simulink model "model_u2_x2"  (R2023b)
settings: Solver=VariableStepAuto  StartTime=0.0  StopTime=100.0  RelTol=1e-3
undefined symbols (not defined in the file or in its folder): a, alfa, beta, K, k, m, w_0, x_0, x_prim_0
settings Model: Creator=student  LastModifiedBy=Jakub

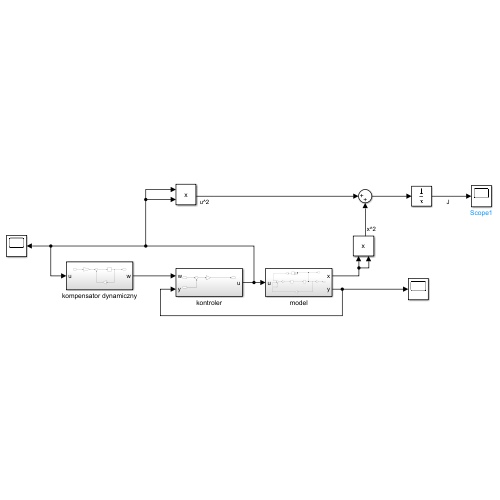
[thumbnail: Simulink's stored preview of the top-level diagram]
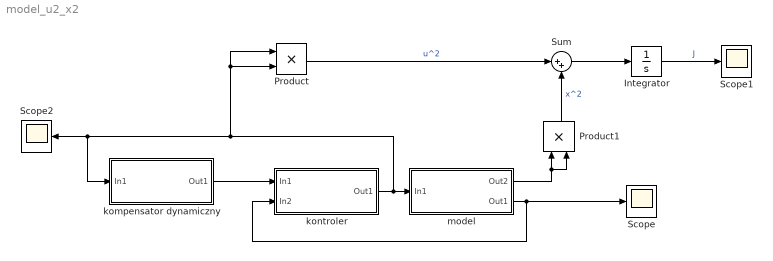
== system model_u2_x2 ==
  Integrator : Integrator
  Product : Product
  Product1 : Product
  Scope : Scope
  Scope1 : Scope
  Scope2 : Scope
  Sum : Sum  Inputs=|++
  kompensator dynamiczny : Subsystem
  kontroler : Subsystem
  model : Subsystem
  wires:
  model/2(Out1) -> Scope/1, kontroler/2(In2)
  kompensator dynamiczny/1(Out1) -> kontroler/1(In1)
  kontroler/1(Out1) -> Product/2, Product/1, Scope2/1, kompensator dynamiczny/1(In1), model/1(In1)
  Integrator/1 -> Scope1/1  "J"
  model/1(Out2) -> Product1/2, Product1/1
  Product1/1 -> Sum/2  "x^2"
  Product/1 -> Sum/1  "u^2"
  Sum/1 -> Integrator/1

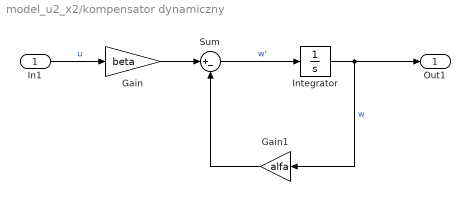
== system model_u2_x2/kompensator dynamiczny ==
  In1 : Inport
  Gain : Gain  Gain=beta
  Gain1 : Gain  Gain=alfa
  Integrator : Integrator  InitialCondition=w_0
  Sum : Sum  Inputs=|+-
  Out1 : Outport
  wires:
  In1/1 -> Gain/1  "u"
  Gain/1 -> Sum/1
  Integrator/1 -> Out1/1, Gain1/1  "w"
  Gain1/1 -> Sum/2
  Sum/1 -> Integrator/1  "w'"

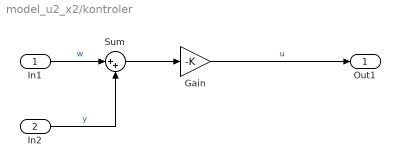
== system model_u2_x2/kontroler ==
  In1 : Inport
  In2 : Inport  Port=2
  Gain : Gain  Gain=-K
  Sum : Sum  Inputs=|++
  Out1 : Outport
  wires:
  Sum/1 -> Gain/1
  In1/1 -> Sum/1  "w"
  In2/1 -> Sum/2  "y"
  Gain/1 -> Out1/1  "u"

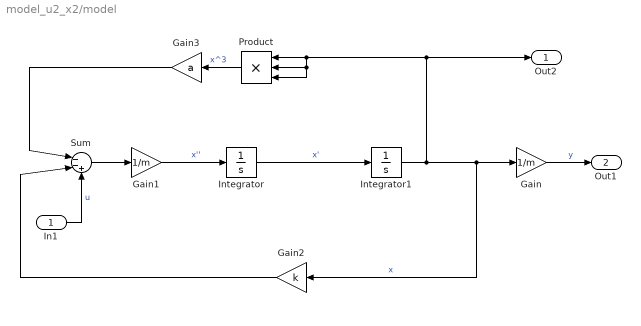
== system model_u2_x2/model ==
  In1 : Inport
  Gain : Gain  Gain=1/m
  Gain1 : Gain  Gain=1/m
  Gain2 : Gain  Gain=k
  Gain3 : Gain  Gain=a
  Integrator : Integrator  InitialCondition=x_prim_0
  Integrator1 : Integrator  InitialCondition=x_0
  Product : Product  Inputs=3
  Sum : Sum  Inputs=|--+
  Out2 : Outport
  Out1 : Outport  Port=2
  wires:
  Gain1/1 -> Integrator/1  "x''"
  Integrator/1 -> Integrator1/1  "x'"
  Integrator1/1 -> Out2/1, Product/3, Product/2, Product/1, Gain2/1, Gain/1  "x"
  Gain/1 -> Out1/1  "y"
  Sum/1 -> Gain1/1
  Gain2/1 -> Sum/2
  Product/1 -> Gain3/1  "x^3"
  Gain3/1 -> Sum/1
  In1/1 -> Sum/3  "u"
